simulink model "twomass (1)"  (R2022b)
settings: Solver=FixedStepAuto  StartTime=0.0  StopTime=10  FixedStep=.05  RelTol=1e-3
values from neighbouring files (symbols this model uses):
  c = 0.8    [CORRECTED_HW_13_4.m]    (also in CORRECTED_HW_14_3.m; Final_Project_State_Space.m = 10; Homework13_4.m; twomassdata.m)
  k1 = 18    [CORRECTED_HW_13_4.m]    (also in CORRECTED_HW_14_3.m; Final_Project_State_Space.m = 13650; Homework13_4.m; twomassdata.m)
  k2 = 21    [CORRECTED_HW_13_4.m]    (also in CORRECTED_HW_14_3.m; Final_Project_State_Space.m = 13650; Homework13_4.m; twomassdata.m)
  m1 = 1    [CORRECTED_HW_13_4.m]    (also in CORRECTED_HW_14_3.m; Final_Project_State_Space.m = 3000; Homework13_4.m; twomassdata.m)
  m2 = 1.4    [CORRECTED_HW_13_4.m]    (also in CORRECTED_HW_14_3.m; Final_Project_State_Space.m = 12000; Homework13_4.m; twomassdata.m)
settings Model: Creator=dherrin  LastModifiedBy=dherrin

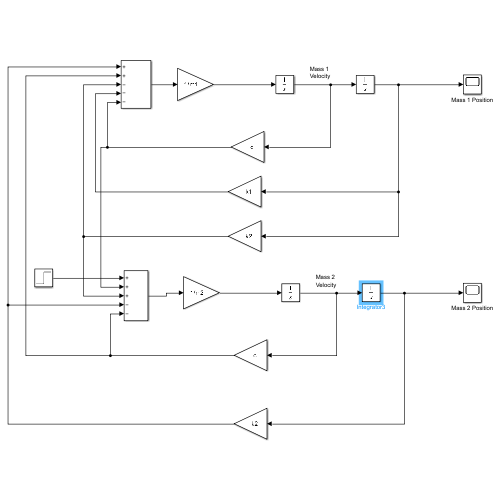
[thumbnail: Simulink's stored preview of the top-level diagram]
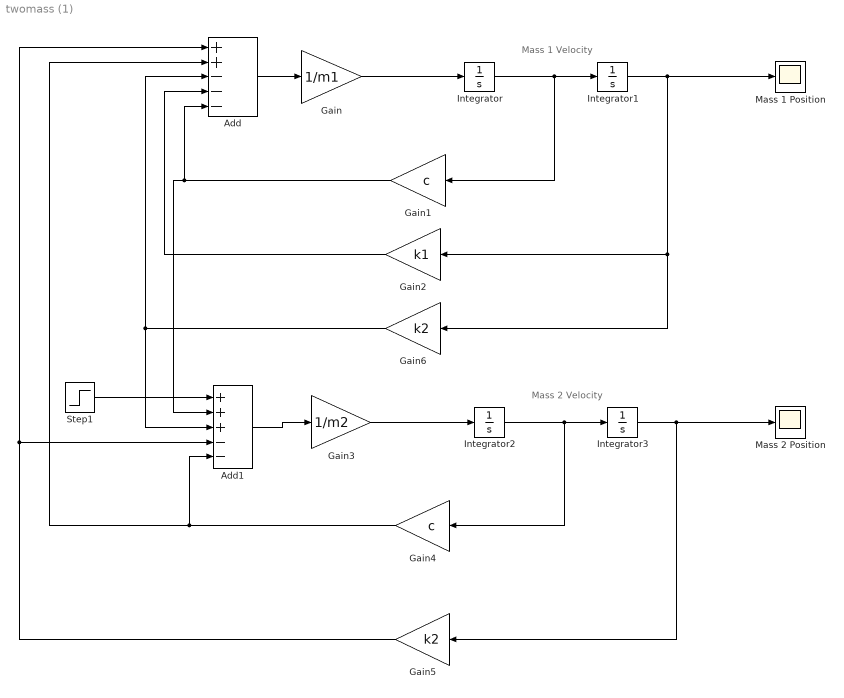
== system twomass (1) ==
  note: Mass 1
      | Velocity
  note: Mass 2
      | Velocity
  Add : Sum  Inputs=++---
  Add1 : Sum  Inputs=+++--
  Gain : Gain  Gain=1/m1
  Gain1 : Gain  Gain=c
  Gain2 : Gain  Gain=k1
  Gain3 : Gain  Gain=1/m2
  Gain4 : Gain  Gain=c
  Gain5 : Gain  Gain=k2
  Gain6 : Gain  Gain=k2
  Integrator : Integrator
  Integrator1 : Integrator  InitialCondition=0.1
  Integrator2 : Integrator
  Integrator3 : Integrator  InitialCondition=-0.1
  Mass 1 Position : Scope
  Mass 2 Position : Scope
  Step1 : Step  Time=0  After=0  SampleTime=0
  wires:
  Gain/1 -> Integrator/1
  Integrator/1 -> Gain1/1, Integrator1/1
  Integrator1/1 -> Gain6/1, Gain2/1, Mass 1 Position/1
  Add/1 -> Gain/1
  Gain2/1 -> Add/4
  Gain4/1 -> Add1/5, Add/2
  Add1/1 -> Gain3/1
  Integrator2/1 -> Gain4/1, Integrator3/1
  Gain5/1 -> Add/1, Add1/4
  Step1/1 -> Add1/1
  Integrator3/1 -> Gain5/1, Mass 2 Position/1
  Gain3/1 -> Integrator2/1
  Gain6/1 -> Add1/3, Add/3
  Gain1/1 -> Add1/2, Add/5
